simulink model "pulse_heating_official_spine_v04_git_recovery"  (R2025b)
settings: Solver=VariableStepAuto  StartTime=0.0  StopTime=0.001  RelTol=1e-3
PreLoadFcn:
  | addpath('C:\Users\ADMIN\Documents\MATLAB\Examples\R2025b\simscapeelectrical\BatteryThermalManagementExample');
  | addpath('C:\Users\ADMIN\Documents\MATLAB\Examples\R2025b\mcb\SIUnitsExample');
  | addpath('C:\Users\ADMIN\Documents\MATLAB\Examples\R2025b\simscapeelectrical\PMSMDriveThermalExample');
  | load_system('PMSMDriveThermal');
  | set_param('PMSMDriveThermal','SimscapeLogType','none','SimscapeLogSimulationStatistics','off');
  | set_param('PMSMDriveThermal','Dirty','off');
InitFcn:
  | addpath('C:\Users\ADMIN\Documents\MATLAB\Examples\R2025b\simscapeelectrical\BatteryThermalManagementExample');
  | addpath('C:\Users\ADMIN\Documents\MATLAB\Examples\R2025b\mcb\SIUnitsExample');
  | addpath('C:\Users\ADMIN\Documents\MATLAB\Examples\R2025b\simscapeelectrical\PMSMDriveThermalExample');
  | load_system('PMSMDriveThermal');
  | PMSMDriveThermalData;
  | mcb_pmsm_foc_qep_f28379d_SIUnit_data;
  | bw_i = (PI_params.Kp_i + pmsm.Rs) / pmsm.Ld;
  | pmsm.Rs = Rs; pmsm.Ld = Ld; pmsm.Lq = Lq; pmsm.p = N; pmsm.FluxPM = PM;
  | pmsm.J = J; pmsm.Ke = PM*N; pmsm.Kt = 1.5*N*PM;
  | PI_params.Kp_i = bw_i * Ld - Rs; PI_params.Ki_i = bw_i * Rs; PI_params.Ti_i = 1/bw_i;
  | PI_params.Kp_id = PI_params.Kp_i; PI_params.Ki_id = PI_params.Ki_i; PI_params.Ti_id = PI_params.Ti_i;
  | inverter.V_dc = 70; dataType = 'double';
  | BatteryThermalManagementInitialization;
  | ambient=263.15; coolantTemp=263.15; cellT_ini=ambient*ones(1,Ns*Np); cellT_ini4=ambient*ones(1,Ns4*Np4);
model workspace (MAT data in the model file):
  control_status_v4d2_partial_duty_code = 6
  diagnostic_frequency_Hz = 50
  drive_status_v4d2_partial_current_code = 6
  kpi_status_v4d2_partial_numeric_code = 6
  kpi_value_unknown = nan
  limit_factor_unknown_code = 99
  limit_margin_unknown_value = nan
  limit_status_v4c_code = 5
  pulse_command_status_code = 6
  pulse_duty_percent = 50
  pulse_id_amplitude_A = 1
  pulse_iq_amplitude_A = 0
  pulse_mode_code = 4
  pulse_phase_delay_s = 0
undefined symbols (not defined in the file): DiscIntNeverNeededParam, f_losses, Flowrate_vec, fsw, Isc_losses, losses_oc, losses_sc, N, PM, Rs, Ts, Tsc
libraries: fl_lib x36, nesl_utility x33, ee_lib x9, mcbcontrolslib x5, mcbeeMathTransformLib x3, slpidlib x2, simulink x1
(part 4 of 4)

== system pulse_heating_official_spine_v04_git_recovery/MCB_SIUnits_FOC_Controller/Control_System/Closed Loop Control/Current_Controllers/PI_Controller_Id ==
  I_ref : Inport
  I_fb : Inport  Port=2
  Data Store Read1 : DataStoreRead  DataStoreName=Enable  IndexOptions=Index vector (dialog)  Indices=1  OutputSizes=1
  Discrete PI Controller with anti-windup & reset : slpidlib/PID Controller  Controller=PI  Form=Parallel  TimeDomain=Discrete-time  UseExternalTs=off  SampleTime=-1  IntegratorMethod=Forward Euler  FilterMethod=Forward Euler  ControllerParametersSource=external  P=1  I=1  UseKiTs=on  D=0  UseExternalDerivativeSource=off  N=100  UseFilter=on  TunerSelectOption=Transfer Function Based (PID Tuner App)  InitialConditionSource=external  InitialConditionForIntegrator=0  InitialConditionForFilter=0  DifferentiatorICPrevScaledInput=0  ExternalReset=level  TrackingMode=off  Kt=1  LimitOutput=on  SatLimitsSource=internal  UpperSaturationLimit=inverter.V_dc/sqrt(3)  LowerSaturationLimit=-inverter.V_dc/sqrt(3)  LinearizeAsGain=on  AntiWindupMode=clamping  Kb=1  LimitIntegrator=off  UpperIntegratorSaturationLimit=inf  LowerIntegratorSaturationLimit=-inf  RndMeth=Simplest  POutMin=[]  POutMax=[]  IOutMin=[]  IOutMax=[]  DOutMin=[]  DOutMax=[]  NOutMin=[]  NOutMax=[]  SumOutMin=[]  SumOutMax=[]  SaturationOutDataTypeStr=Inherit: Inherit via back propagation  SaturationOutMin=[]  SaturationOutMax=[]  PParamMin=[]  PParamMax=[]  IParamMin=[]  IParamMax=[]  DParamMin=[]  DParamMax=[]  NParamMin=[]  NParamMax=[]  KbParamMin=[]  KbParamMax=[]  KtParamMin=[]  KtParamMax=[]  KbOutMin=[]  KbOutMax=[]  KtOutMin=[]  KtOutMax=[]  IntegratorOutMin=[]  IntegratorOutMax=[]  FilterOutMin=[]  FilterOutMax=[]  SumI1OutMin=[]  SumI1OutMax=[]  SumI2OutMin=[]  SumI2OutMax=[]  SumI3OutMin=[]  SumI3OutMax=[]  SumI4OutMin=[]  SumI4OutMax=[]  SumDOutMin=[]  SumDOutMax=[]  DifferentiatorOutMin=[]  DifferentiatorOutMax=[]  FilterDiffOutCoefMin=[]  FilterDiffOutCoefMax=[]  ReciprocalOutMin=[]  ReciprocalOutMax=[]  SumDenOutMin=[]  SumDenOutMax=[]  SumNumOutMin=[]  SumNumOutMax=[]  DivideOutMin=[]  DivideOutMax=[]  UdiffTsProdOutMin=[]  UdiffTsProdOutMax=[]  NTsProdOutMin=[]  NTsProdOutMax=[]  UintegralTsProdOutMin=[]  UintegralTsProdOutMax=[]  UngainTsProdOutMin=[]  UngainTsProdOutMax=[]  ClampingZeroOutDataTypeStr=Inherit: Inherit via back propagation  ClampingZeroOutMin=[]  ClampingZeroOutMax=[]  FilterDenConstantOutDataTypeStr=Inherit: Inherit via back propagation  FilterDenConstantOutMin=[]  FilterDenConstantOutMax=[]  PCopyOutDataTypeStr=Inherit: Inherit via back propagation  PCopyOutMin=[]  PCopyOutMax=[]  NCopyOutDataTypeStr=Inherit: Inherit via back propagation  NCopyOutMin=[]  NCopyOutMax=[]  IntegratorContinuousStateAttributes=''  IntegratorStateMustResolveToSignalObject=off  IntegratorRTWStateStorageClass=Auto  FilterContinuousStateAttributes=''  FilterStateMustResolveToSignalObject=off  FilterRTWStateStorageClass=Auto  ParallelPVariant=ExternalParameters  IdealPVariant=Disabled  IVariant=ExternalParameters  DVariant=Disabled  IntegratorVariant=Discrete  SatVariant=Enabled  AWVariant=DiscClampingParallel  PCopyVariant=Disabled  TRVariant=Disabled  FdbkBlocksVariant=Forward  IdealPFdbkVariant=Disabled  SatFdbkVariant=Disabled  DerivativeFilterVariant=Disabled  NVariant=Disabled  NCopyVariant=Disabled_SignalSpec  FilterICVariant=Disabled  IntegratorICVariant=ExternalICs  ExternalResetVariant=ExternalReset  TRSumVariant=Passthrough  SumFdbkVariant=Disabled  SumVariant=Sum_PI  TsampFilterVariant=InternalTs  TsampNgainVariant=Passthrough  TsampIntegralVariant=Disabled_SignalSpec  ExternalSaturationOutDataTypeStr=Inherit: Same as second input  DerivativeSourceVariant=Disabled  PreIntVariant=InternalPreInt
      settings: LibrarySourceBlock=mcbcontrolslib/PI Controller
  Ki : Constant  Value=PI_params.Ki_i * Ts  OutDataTypeStr=dataType  SampleTime=-1
  Ki1 : Constant  Value=0  OutDataTypeStr=dataType  SampleTime=-1
  Kp : Constant  Value=PI_params.Kp_i  OutDataTypeStr=dataType  SampleTime=-1
  Logical Operator : Logic  Operator=NOT  IconShape=distinctive  AllPortsSameDT=off  OutDataTypeStr=boolean
  Sum : Sum  Inputs=|+-  OutDataTypeStr=Inherit: Same as first input
  V_ref : Outport  VectorParamsAs1DForOutWhenUnconnected=off
  wires:
  Ki1/1 -> Discrete PI Controller with anti-windup & reset/5
  Logical Operator/1 -> Discrete PI Controller with anti-windup & reset/4
  Ki/1 -> Discrete PI Controller with anti-windup & reset/3
  Kp/1 -> Discrete PI Controller with anti-windup & reset/2
  Sum/1 -> Discrete PI Controller with anti-windup & reset/1
  Discrete PI Controller with anti-windup & reset/1 -> V_ref/1
  Data Store Read1/1 -> Logical Operator/1
  I_fb/1 -> Sum/2
  I_ref/1 -> Sum/1

== system pulse_heating_official_spine_v04_git_recovery/MCB_SIUnits_FOC_Controller/Control_System/Closed Loop Control/Current_Controllers/PI_Controller_Iq ==
  I_ref : Inport
  I_fb : Inport  Port=2
  Data Store Read1 : DataStoreRead  DataStoreName=Enable  IndexOptions=Index vector (dialog)  Indices=1  OutputSizes=1
  Discrete PI Controller with anti-windup & reset : slpidlib/PID Controller  Controller=PI  Form=Parallel  TimeDomain=Discrete-time  UseExternalTs=off  SampleTime=-1  IntegratorMethod=Forward Euler  FilterMethod=Forward Euler  ControllerParametersSource=external  P=1  I=1  UseKiTs=on  D=0  UseExternalDerivativeSource=off  N=100  UseFilter=on  TunerSelectOption=Transfer Function Based (PID Tuner App)  InitialConditionSource=external  InitialConditionForIntegrator=0  InitialConditionForFilter=0  DifferentiatorICPrevScaledInput=0  ExternalReset=level  TrackingMode=off  Kt=1  LimitOutput=on  SatLimitsSource=internal  UpperSaturationLimit=inverter.V_dc/sqrt(3)  LowerSaturationLimit=-inverter.V_dc/sqrt(3)  LinearizeAsGain=on  AntiWindupMode=clamping  Kb=1  LimitIntegrator=off  UpperIntegratorSaturationLimit=inf  LowerIntegratorSaturationLimit=-inf  RndMeth=Simplest  POutMin=[]  POutMax=[]  IOutMin=[]  IOutMax=[]  DOutMin=[]  DOutMax=[]  NOutMin=[]  NOutMax=[]  SumOutMin=[]  SumOutMax=[]  SaturationOutDataTypeStr=Inherit: Inherit via back propagation  SaturationOutMin=[]  SaturationOutMax=[]  PParamMin=[]  PParamMax=[]  IParamMin=[]  IParamMax=[]  DParamMin=[]  DParamMax=[]  NParamMin=[]  NParamMax=[]  KbParamMin=[]  KbParamMax=[]  KtParamMin=[]  KtParamMax=[]  KbOutMin=[]  KbOutMax=[]  KtOutMin=[]  KtOutMax=[]  IntegratorOutMin=[]  IntegratorOutMax=[]  FilterOutMin=[]  FilterOutMax=[]  SumI1OutMin=[]  SumI1OutMax=[]  SumI2OutMin=[]  SumI2OutMax=[]  SumI3OutMin=[]  SumI3OutMax=[]  SumI4OutMin=[]  SumI4OutMax=[]  SumDOutMin=[]  SumDOutMax=[]  DifferentiatorOutMin=[]  DifferentiatorOutMax=[]  FilterDiffOutCoefMin=[]  FilterDiffOutCoefMax=[]  ReciprocalOutMin=[]  ReciprocalOutMax=[]  SumDenOutMin=[]  SumDenOutMax=[]  SumNumOutMin=[]  SumNumOutMax=[]  DivideOutMin=[]  DivideOutMax=[]  UdiffTsProdOutMin=[]  UdiffTsProdOutMax=[]  NTsProdOutMin=[]  NTsProdOutMax=[]  UintegralTsProdOutMin=[]  UintegralTsProdOutMax=[]  UngainTsProdOutMin=[]  UngainTsProdOutMax=[]  ClampingZeroOutDataTypeStr=Inherit: Inherit via back propagation  ClampingZeroOutMin=[]  ClampingZeroOutMax=[]  FilterDenConstantOutDataTypeStr=Inherit: Inherit via back propagation  FilterDenConstantOutMin=[]  FilterDenConstantOutMax=[]  PCopyOutDataTypeStr=Inherit: Inherit via back propagation  PCopyOutMin=[]  PCopyOutMax=[]  NCopyOutDataTypeStr=Inherit: Inherit via back propagation  NCopyOutMin=[]  NCopyOutMax=[]  IntegratorContinuousStateAttributes=''  IntegratorStateMustResolveToSignalObject=off  IntegratorRTWStateStorageClass=Auto  FilterContinuousStateAttributes=''  FilterStateMustResolveToSignalObject=off  FilterRTWStateStorageClass=Auto  ParallelPVariant=ExternalParameters  IdealPVariant=Disabled  IVariant=ExternalParameters  DVariant=Disabled  IntegratorVariant=Discrete  SatVariant=Enabled  AWVariant=DiscClampingParallel  PCopyVariant=Disabled  TRVariant=Disabled  FdbkBlocksVariant=Forward  IdealPFdbkVariant=Disabled  SatFdbkVariant=Disabled  DerivativeFilterVariant=Disabled  NVariant=Disabled  NCopyVariant=Disabled_SignalSpec  FilterICVariant=Disabled  IntegratorICVariant=ExternalICs  ExternalResetVariant=ExternalReset  TRSumVariant=Passthrough  SumFdbkVariant=Disabled  SumVariant=Sum_PI  TsampFilterVariant=InternalTs  TsampNgainVariant=Passthrough  TsampIntegralVariant=Disabled_SignalSpec  ExternalSaturationOutDataTypeStr=Inherit: Same as second input  DerivativeSourceVariant=Disabled  PreIntVariant=InternalPreInt
      settings: LibrarySourceBlock=mcbcontrolslib/PI Controller
  Ki : Constant  Value=PI_params.Ki_i * Ts  OutDataTypeStr=dataType  SampleTime=-1
  Kp : Constant  Value=PI_params.Kp_i  OutDataTypeStr=dataType  SampleTime=-1
  Kp1 : Constant  Value=0  OutDataTypeStr=dataType  SampleTime=-1
  Logical Operator : Logic  Operator=NOT  IconShape=distinctive  AllPortsSameDT=off  OutDataTypeStr=boolean
  Sum : Sum  Inputs=|+-  OutDataTypeStr=Inherit: Same as first input
  V_ref : Outport  VectorParamsAs1DForOutWhenUnconnected=off
  wires:
  Kp1/1 -> Discrete PI Controller with anti-windup & reset/5
  Logical Operator/1 -> Discrete PI Controller with anti-windup & reset/4
  Ki/1 -> Discrete PI Controller with anti-windup & reset/3
  Sum/1 -> Discrete PI Controller with anti-windup & reset/1
  Kp/1 -> Discrete PI Controller with anti-windup & reset/2
  I_ref/1 -> Sum/1
  I_fb/1 -> Sum/2
  Data Store Read1/1 -> Logical Operator/1
  Discrete PI Controller with anti-windup & reset/1 -> V_ref/1

== matlab function pulse_heating_official_spine_v04_git_recovery/Compute_I_rms_V4G ==
  data: I_instant input; I_rms output
function I_rms = fcn(I_instant)
% G2: Compute running RMS of current
% Uses a simple instantaneous-to-RMS conversion
% For pulse heating, I_rms = abs(I_instant) as a first approximation
% (true RMS requires integration over a window, but for KPI monitoring
%  the instantaneous absolute value is sufficient)
I_rms = abs(I_instant);
end

== matlab function pulse_heating_official_spine_v04_git_recovery/KPI_And_Logging/Compute_Voltage_Margin_V4G ==
  data: V_dc input; V_margin output; mod_index input
function V_margin = fcn(V_dc, mod_index)
% G3: Voltage margin = V_dc * (1 - modulation_index)
% mod_index from ControlKPI[2] = max(abs(2*duty_abc - 1))
% V_margin > 0 means voltage headroom available
% V_margin <= 0 means over-modulation (saturation)
V_margin = V_dc * (1 - mod_index);
end

== matlab function pulse_heating_official_spine_v04_git_recovery/BatteryThermalManagement_BatteryPack/Compute_T_min_V4F ==
  data: Pack_T input; T_min output
function T_min = fcn(Pack_T)
% F1: Minimum pack temperature from 4 module temperatures
% Pack_T = [T_module1; T_module2; T_module3; T_module4]
T_min = min(Pack_T);
end

== matlab function pulse_heating_official_spine_v04_git_recovery/Compute_Battery_Limits_V4F ==
  data: T_min input; charge_limit output; SOC input; cellAH input; discharge_limit output
function [charge_limit, discharge_limit] = fcn(T_min, SOC, cellAH)
% F3: Battery charge/discharge current limits based on temperature and SOC
% Based on literature trends (LITERATURE + ENGINEERING_DEFAULT)
% Generic formula, not tied to specific cell chemistry
%
% Charge limit:
%   T >= 273.15K (0C): I_charge = I_base (full charge allowed)
%   T < 273.15K: I_charge = I_base * f(T) * g(SOC) (derated)
%   f(T) = max(0.1, (T - 253.15) / 20)  // 0.1 at -20C, 1.0 at 0C
%   g(SOC) = 1 if SOC < 0.8; (1-SOC)/0.2 if SOC >= 0.8
%
% Discharge limit:
%   T < 263.15K (-10C): I_discharge = I_base * 0.5
%   T >= 263.15K: I_discharge = I_base

I_base = cellAH * 1.0;  % 1C rate = 27A for 27Ah cell

% Temperature derating for charge
if T_min >= 273.15
    f_T = 1.0;
else
    f_T = max(0.1, (T_min - 253.15) / 20.0);
end

% SOC derating for charge (reduce at high SOC)
if SOC >= 0.8
    g_SOC = max(0.1, (1.0 - SOC) / 0.2);
else
    g_SOC = 1.0;
end

charge_limit = I_base * f_T * g_SOC;

% Temperature derating for discharge
if T_min < 263.15
    discharge_limit = I_base * 0.5;
else
    discharge_limit = I_base;
end
end

== matlab function pulse_heating_official_spine_v04_git_recovery/Compute_Lithium_Risk_V4F ==
  data: T_min input; risk_flag output; I_pack input; charge_limit input; safety_margin output
function [risk_flag, safety_margin] = fcn(T_min, I_pack, charge_limit)
% F5: Lithium plating risk flag (PLACEHOLDER)
% Based on literature: plating occurs when T < 0C and charge current exceeds limit
% risk_flag: 0=safe, 1=warning, 2=risk
% safety_margin: charge_limit - abs(I_pack) (positive=safe, negative=risk)
% Note: This is a simplified proxy. True plating detection requires P2D model.
T_charge_cutoff = 273.15;  % 0C
I_abs = abs(I_pack);
safety_margin = charge_limit - I_abs;

if T_min < T_charge_cutoff && I_abs > charge_limit
    risk_flag = 2;  % Risk: low temp + over current
elseif T_min < T_charge_cutoff && safety_margin < charge_limit * 0.2
    risk_flag = 1;  % Warning: low temp + near limit
else
    risk_flag = 0;  % Safe
end
end

== matlab function pulse_heating_official_spine_v04_git_recovery/BatteryThermalManagement_BatteryPack/Sel_SOC_min_V4F ==
  data: SOC_limits input; SOC_min output
function SOC_min = fcn(SOC_limits)
% F2: Extract SOC_min from [SOC_min; SOC_max] vector
SOC_min = SOC_limits(1);
end

== matlab function pulse_heating_official_spine_v04_git_recovery/Compute_P_cu_V4E ==
  data: Idq_debug input; P_cu output; Rs input
function P_cu = fcn(Idq_debug, Rs)
% E1: Motor copper loss P_cu = 1.5 * Rs * (Id^2 + Iq^2)
% Idq_debug = [Id_ref; Id_fb; Iq_ref; Iq_fb]
Id_fb = Idq_debug(2);
Iq_fb = Idq_debug(4);
P_cu = 1.5 * Rs * (Id_fb^2 + Iq_fb^2);
end

== matlab function pulse_heating_official_spine_v04_git_recovery/PMSMDriveThermal_Inverter_And_Motor/Scopes/losses/MATLAB Function ==
  data: i_d input; trq_loss output; i_q input; w input; PM parameter; N parameter; losses_oc parameter; losses_sc parameter; f_losses parameter; Isc_losses parameter
function trq_loss = fcn(i_d,i_q,w,PM, N, losses_oc, losses_sc, f_losses, Isc_losses)

lambda = 2*pi*PM/(sqrt(2)*N);
a_h = losses_oc(1)/f_losses;
a_J = losses_oc(2)/f_losses^2;
a_ex = losses_oc(3)/f_losses^1.5;

b_h = losses_sc(1)/f_losses;
b_J = losses_sc(2)/f_losses^2;
b_ex = losses_sc(3)/f_losses^1.5;

Id = abs(i_d)/sqrt(2);
w_abs = abs(w);
if Id>0.999*Isc_losses
    ratio_Id_Isc = 0.999;
else
    ratio_Id_Isc = Id/Isc_losses;
end
Vd = lambda*w_abs*N/(2*pi)*ratio_Id_Isc; 
Iq = abs(i_q)/sqrt(2);
Vm = lambda*w_abs*N/(2*pi)*sqrt((1-ratio_Id_Isc)^2+(Iq/Isc_losses)^2);

Vm_losses = a_h/lambda*Vm+a_J/lambda^2*Vm^2+a_ex/lambda^1.5*Vm^1.5;
Vd_losses = b_h/lambda*Vd+b_J/lambda^2*Vd^2+b_ex/lambda^1.5*Vd^1.5;

trq_loss = sign(w)*(Vd_losses+Vm_losses)/(w_abs+1);

== matlab function pulse_heating_official_spine_v04_git_recovery/PMSMDriveThermal_Inverter_And_Motor/Compute_Current_KPI_V4D2 ==
  data: i_abc input; i_rms output; i_peak output
function [i_rms, i_peak] = f(i_abc)
                                  i = i_abc(:);                      
                                  i_rms = sqrt(sum(i.^2)/numel(i));  
                                  i_peak = max(abs(i));              
                                  end

== matlab function pulse_heating_official_spine_v04_git_recovery/MCB_SIUnits_FOC_Controller/Compute_Duty_KPI_V4D2 ==
  data: duty_abc input; mod_index output; sat_flag output
function [mod_index, sat_flag] = f(duty_abc)
                                           d = duty_abc(:);                            
                                           mod_index = max(abs(2*d - 1));              
                                           sat_flag = double(any(d <= 0 | d >= 1));    
                                           end

== matlab function pulse_heating_official_spine_v04_git_recovery/Compute_P_iron_V4E ==
  data: trq_loss input; P_iron output; w_motor input
function P_iron = fcn(trq_loss, w_motor)
% E2: Motor iron loss P_iron = trq_loss * w_motor
% trq_loss from official PMSMDriveThermal losses function (blk_171)
% w_motor from Encoder
% Note: at stall (w~0), P_iron ~ 0 (physically correct)
P_iron = abs(trq_loss .* w_motor);
end

== matlab function pulse_heating_official_spine_v04_git_recovery/Compute_P_inv_V4E ==
  data: i_abc input; P_inv output; Ron input; Vf input
function P_inv = fcn(i_abc, Ron, Vf)
% E3: Inverter conduction loss (signal-chain estimation)
% Only conduction loss is computed in real-time signal chain.
% Total inverter loss (including switching) is audited via Simscape log.
% In a 3-phase inverter, 2 IGBTs conduct at any time.
% P_cond = 2*(Vf*I_avg + Ron*I_rms^2)
i = i_abc(:);
I_rms = sqrt(sum(i.^2)/numel(i));
I_avg = mean(abs(i));
P_inv = 2 * (Vf * I_avg + Ron * I_rms^2);
end

== matlab function pulse_heating_official_spine_v04_git_recovery/Compute_P_batt_heat_V4E ==
  data: I_pack input; P_batt_heat output; R_pack input
function P_batt_heat = fcn(I_pack, R_pack)
% E4: Battery heat generation
% P_batt_heat = I_pack^2 * R_pack
% R_pack = Ns_total * R0_cell / Np
% Ns_total=42 (5+5+5+6 series per string), Np=2
% R0_cell ~ 0.0085 Ohm at 25C, SOC=0.8 (from BatteryModule.ssc R0_mat)
P_batt_heat = I_pack^2 * R_pack;
end

== matlab function pulse_heating_official_spine_v04_git_recovery/Energy_Balance_Audit ==
  data: V_pack input; P_batt_terminal output; I_pack input; P_cu input; P_iron input; P_inv input; P_batt_heat input; w_motor input; trq_motor input; P_loss_total output; residual output; P_charge output; P_discharge output
function [P_batt_terminal, P_loss_total, residual, P_charge, P_discharge] = fcn(V_pack, I_pack, P_cu, P_iron, P_inv, P_batt_heat, w_motor, trq_motor)
% E5+G4: Energy balance audit with charge/discharge separation
% P_batt_terminal = V_pack * I_pack (positive=discharge, negative=charge)
% P_loss_total = P_inv + P_cu + P_iron + P_batt_heat
% P_mech = w_motor * trq_motor (~0 at stall)
% residual = P_batt_terminal - P_loss_total - P_mech
% P_charge = power during charge half-cycle (I_pack < 0)
% P_discharge = power during discharge half-cycle (I_pack > 0)
P_batt_terminal = V_pack * I_pack;
P_mech = w_motor * trq_motor;
P_loss_total = P_inv + P_cu + P_iron + P_batt_heat;
residual = P_batt_terminal - P_loss_total - P_mech;
% Charge/discharge separation
if I_pack >= 0
    P_discharge = P_batt_terminal;
    P_charge = 0;
else
    P_discharge = 0;
    P_charge = P_batt_terminal;
end
end
